simulink model "WPL_APA_parallel"  (R2020b)
settings: Solver=FixedStepAuto  StartTime=0.0  StopTime=inf  FixedStep=0.02  RelTol=1e-3
undefined symbols (not defined in the file): Drive, Steer
libraries: robotlib x10, simulink x1
(part 3 of 3)

== matlab function WPL_APA_parallel/Planner and Controller/Subsystem/MATLAB Function ==
  data: Xr input; v_des output; Yr input; Yaw input; xd input; yd input; thetad input; V input; deltad input; U1 input; delta_des output; delta_t output; fval output; exitflag output; U2 input; U1_ output; U2_ output
function [v_des,delta_des,delta_t,fval,exitflag,U1_,U2_] = fcn(Xr,Yr,Yaw,xd,yd,thetad,V,deltad,U1,U2)
    tstart=tic;
    Nx=3;%状态量的个数
    Nu =2;%控制量的个数
    Np =30;%预测步长Np =60;20
    Nc=1;%控制步长Nc=30;1
    Row=10;%松弛因子
    t_d =Yaw;%t_d =Yaw*pi/180
    
    r=zeros(3,1);
    r(1)=xd;
    r(2)=yd;
    r(3)=thetad;
    vd1=V;
    vd2=deltad;

    kesi=zeros(Nx+Nu,1);
    kesi(1)=Xr-r(1);%Xr==X(1)
    kesi(2)=Yr-r(2);%Yr==X(2)
    kesi(3)=t_d-r(3); %Yaw==X(3)
    kesi(4)=U1;
    kesi(5)=U2;

    T=0.1;
    L = 1.88;

%矩阵初始化   
    u_piao=zeros(Nx,Nu);
    Q=100*eye(Nx*Np,Nx*Np);    
    R=5*eye(Nu*Nc);
    a=[1    0   -vd1*sin(t_d)*T;
       0    1   vd1*cos(t_d)*T;
       0    0   1];
    b=[cos(t_d)*T   0;
       sin(t_d)*T   0;
       tan(vd2)*T/L      vd1*T/(cos(vd2)^2)];%%%%%%%%%%%%%%%%%%%%%%%tan(vd2)*T/L vd1*T/(cos(vd2)^2)%%%%%%%%%
%     A_cell=cell(2,2);
%     B_cell=cell(2,1);
%     A_cell{1,1}=a;
%     A_cell{1,2}=b;
%     A_cell{2,1}=zeros(Nu,Nx);
%     A_cell{2,2}=eye(Nu);
%     B_cell{1,1}=b;
%     B_cell{2,1}=eye(Nu);
%     A=cell2mat(A_cell);
%     B=cell2mat(B_cell);
    A=[a,b;
       zeros(Nu,Nx),eye(Nu)];
    B=[b;eye(Nu)];
    C=[1 0 0 0 0;0 1 0 0 0;0 0 1 0 0;];
    
    
%     PHI_cell=cell(Np,1);
%     THETA_cell=cell(Np,Nc);
%     for j=1:1:Np
%         PHI_cell{j,1}=C*A^j;
%         for k=1:1:Nc
%             if k<=j
%                 THETA_cell{j,k}=C*A^(j-k)*B;
%             else 
%                 THETA_cell{j,k}=zeros(Nx,Nu);
%             end
%         end
%     end
%     PHI=cell2mat(PHI_cell);%size(PHI)=[Nx*Np Nx+Nu]
%     THETA=cell2mat(THETA_cell);%size(THETA)=[Nx*Np Nu*(Nc+1)]    
%     coder.varsize('PHI',[Np*3,1*5]);
%     coder.varsize('THETA',[Np*Nx,Nc*Nu]);
    coder.varsize('PHI',[100,5]);
    coder.varsize('THETA',[100,5]);
    PHI=C*A;
    THETA=C*A^(1-1)*B;
    for j=2:1:Np
        PHI=[PHI;C*A^j];
        THETA=[THETA;C*A^(j-1)*B];
    end
    
%     H_cell=cell(2,2);
%     H_cell{1,1}=THETA'*Q*THETA+R;
%     H_cell{1,2}=zeros(Nu*Nc,1);
%     H_cell{2,1}=zeros(1,Nu*Nc);
%     H_cell{2,2}=Row;
%     H=cell2mat(H_cell);
    error=PHI*kesi;
%     f_cell=cell(1,2);
%     f_cell{1,1}=2*error'*Q*THETA;
%     f_cell{1,2}=0;
%     f=cell2mat(f_cell); 
    H=[THETA'*Q*THETA+R,zeros(Nu*Nc,1);
        zeros(1,Nu*Nc),Row];
    f=[2*error'*Q*THETA,0];
 %% 以下为约束生成区域
 %不等式约束
    A_t=zeros(Nc,Nc);%见falcone论文 P181
    for p=1:1:Nc
        for q=1:1:Nc
            if q<=p 
                A_t(p,q)=1;
            else 
                A_t(p,q)=0;
            end
        end 
    end 
    A_I=kron(A_t,eye(Nu));%对应于falcone论文约束处理的矩阵A,求克罗内克积
    Ut=kron(ones(Nc,1),[U1;U2]);%此处感觉论文里的克罗内科积有问题,暂时交换顺序
    umin=[-0.1;-0.1];%维数与控制变量的个数相同
    umax=[0.1;0.1];
    delta_umin=[-0.02;-0.02;];%delta_umin=[0.05;-0.0082;];原代码有错，速度变化下界没加负号
    delta_umax=[0.02;0.02];
    Umin=kron(ones(Nc,1),umin);
    Umax=kron(ones(Nc,1),umax);
%     A_cons_cell={A_I zeros(Nu*Nc,1);-A_I zeros(Nu*Nc,1)};
%     b_cons_cell={Umax-Ut;-Umin+Ut};
%     A_cons=cell2mat(A_cons_cell);%（求解方程）状态量不等式约束增益矩阵，转换为绝对值的取值范围
%     b_cons=cell2mat(b_cons_cell);%（求解方程）状态量不等式约束的取值    
    A_cons=[A_I zeros(Nu*Nc,1);-A_I zeros(Nu*Nc,1)];
    b_cons=[Umax-Ut;-Umin+Ut];
    
   % 状态量约束
    M=10; 
    delta_Umin=kron(ones(Nc,1),delta_umin);
    delta_Umax=kron(ones(Nc,1),delta_umax);
    lb=[delta_Umin;0];%（求解方程）状态量下界，包含控制时域内控制增量和松弛因子
    ub=[delta_Umax;M];%（求解方程）状态量上界，包含控制时域内控制增量和松弛因子
    
    %% 开始求解过程
%     opts = optimoptions('quadprog','Algorithm','active-set','OptimalityTolerance',1e-5,'MaxIterations',200);
%     x_start=zeros(Nc+1,1);
%     [du,fval,exitflag]=quadprog(H,f,A_cons,b_cons,[],[],lb,ub,x_start,opts);
    
    opts = optimoptions('quadprog','Algorithm','active-set');
    x_start=zeros(2*Nc+1,1);
    [X,fval,exitflag]=quadprog(H,f,A_cons,b_cons,[],[],lb,ub,x_start,opts);

    %options = optimset('Algorithm','active-set');新版quadprog不能用有效集法，这里选内点法
%     options = optimset('Algorithm','interior-point-convex'); 
%     [X,fval,exitflag]=quadprog(H,f,A_cons,b_cons,[],[],lb,ub,[],options);
    %% 计算输出    
    u_piao(1)=X(1);
    u_piao(2)=X(2);
    U1_=kesi(4)+u_piao(1);%用于存储上一个时刻的控制量
    U2_=kesi(5)+u_piao(2);
    v_des=U1_+vd1;
    delta_des=U2_+vd2;
    delta_t=toc(tstart);

== matlab function WPL_APA_parallel/Planner and Controller/MATLAB Function1 ==
  data: u input; y output
function y = fcn(u)

y = round(u);
